simulink model "Simulate_FFNN"  (Simulink 10.2)
settings: Solver=ode45  StartTime=0.0  StopTime=10  RelTol=1e-3  EnableMultiTasking=on
libraries: slpidlib x22
settings Model: Creator=Administrator  LastModifiedBy=hunter
settings SolverCC: ZeroCrossControl=DisableAll
settings DataIOCC: LimitDataPoints=on
settings OptimizationCC: ExpressionDepthLimit=2147483647
settings DebuggingCC: SolverPrmCheckMsg=warning  StateNameClashWarn=warning

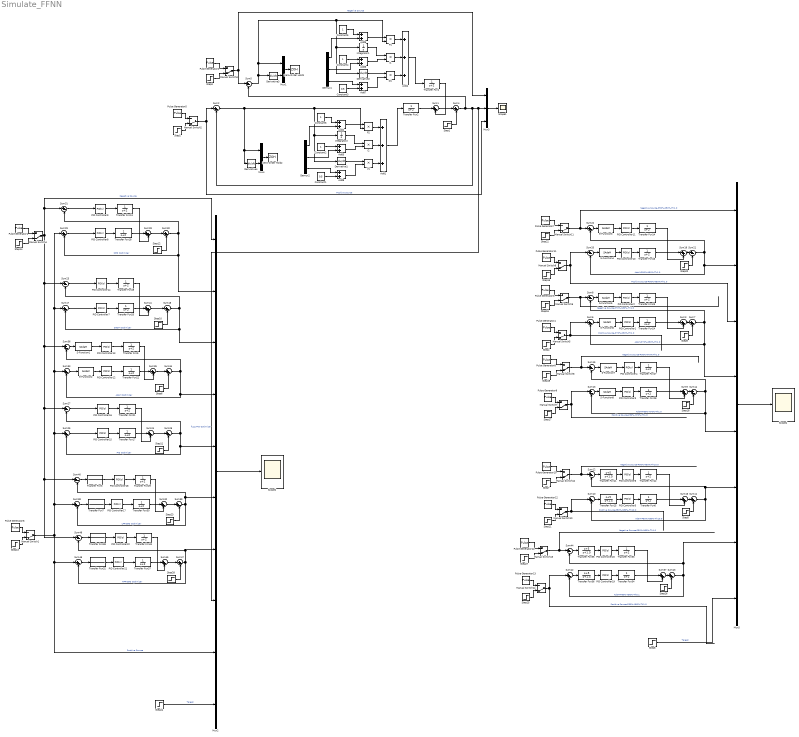
== system Simulate_FFNN ==
  Add1 : Sum  Inputs=+++
  Add{2..3,5..8} (6 alike) : Sum
  Add4 : Sum  Inputs=+++
  Constant1 : Constant  Value=0.5
  Constant{2,4..6} (4 alike) : Constant
  Constant3 : Constant  Value=0.5
  D1 : Product
  D2 : Product
  Demux1 : Demux  Outputs=3
  Demux2 : Demux  Outputs=3
  Derivative{1..4} (4 alike) : Derivative
  I1 : Product
  I2 : Product
  Integrator1 : Integrator
  Integrator2 : Integrator
  Manual Switch{1..14} (14 alike) : ManualSwitch  CurrentSetting=0
  Mux1 : Mux  Inputs=2
  Mux2 : Mux  Inputs=10
  Mux3 : Mux  Inputs=3
  Mux4 : Mux  Inputs=2
  Mux5 : Mux  Inputs=8
  P1 : Product
  P2 : Product
  PID Controller{1..4,8..13,17..18,21..22} (14 alike) : slpidlib/PID Controller  Controller=PID  Form=Parallel  TimeDomain=Continuous-time  UseExternalTs=off  SampleTime=-1  IntegratorMethod=Forward Euler  FilterMethod=Forward Euler  ControllerParametersSource=internal  P=1  I=0  D=0  UseFilter=on  N=100  TunerSelectOption=Transfer Function Based (PID Tuner App)  InitialConditionSource=internal  InitialConditionForIntegrator=0  InitialConditionForFilter=0  DifferentiatorICPrevScaledInput=0  ExternalReset=none  TrackingMode=off  Kt=1  LimitOutput=off  SatLimitsSource=internal  UpperSaturationLimit=inf  LowerSaturationLimit=-inf  LinearizeAsGain=on  AntiWindupMode=none  Kb=1  POutMin=[]  POutMax=[]  IOutMin=[]  IOutMax=[]  DOutMin=[]  DOutMax=[]  NOutMin=[]  NOutMax=[]  SumOutMin=[]  SumOutMax=[]  SaturationOutMin=[]  SaturationOutMax=[]  PParamMin=[]  PParamMax=[]  IParamMin=[]  IParamMax=[]  DParamMin=[]  DParamMax=[]  NParamMin=[]  NParamMax=[]  KbParamMin=[]  KbParamMax=[]  KtParamMin=[]  KtParamMax=[]  KbOutMin=[]  KbOutMax=[]  KtOutMin=[]  KtOutMax=[]  IntegratorOutMin=[]  IntegratorOutMax=[]  FilterOutMin=[]  FilterOutMax=[]  SumI1OutMin=[]  SumI1OutMax=[]  SumI2OutMin=[]  SumI2OutMax=[]  SumI3OutMin=[]  SumI3OutMax=[]  SumI4OutMin=[]  SumI4OutMax=[]  SumDOutMin=[]  SumDOutMax=[]  DifferentiatorOutMin=[]  DifferentiatorOutMax=[]  FilterDiffOutCoefMin=[]  FilterDiffOutCoefMax=[]  ReciprocalOutMin=[]  ReciprocalOutMax=[]  SumDenOutMin=[]  SumDenOutMax=[]  SumNumOutMin=[]  SumNumOutMax=[]  DivideOutMin=[]  DivideOutMax=[]  UdiffTsProdOutMin=[]  UdiffTsProdOutMax=[]  NTsProdOutMin=[]  NTsProdOutMax=[]  UintegralTsProdOutMin=[]  UintegralTsProdOutMax=[]  UngainTsProdOutMin=[]  UngainTsProdOutMax=[]  IntegratorContinuousStateAttributes=''  IntegratorStateMustResolveToSignalObject=off  IntegratorRTWStateStorageClass=Auto  FilterContinuousStateAttributes=''  FilterStateMustResolveToSignalObject=off  FilterRTWStateStorageClass=Auto  ParallelPVariant=InternalParameters  IdealPVariant=Disabled  IVariant=InternalParameters  DVariant=InternalParameters  IntegratorVariant=Continuous  SatVariant=Disabled  AWVariant=Passthrough  PCopyVariant=Disabled  TRVariant=Disabled  FdbkBlocksVariant=Forward  IdealPFdbkVariant=Disabled  SatFdbkVariant=Disabled  DerivativeFilterVariant=ContFilter  NVariant=InternalParameters  NCopyVariant=Disabled  FilterICVariant=InternalICsFilter  IntegratorICVariant=InternalICs  ExternalResetVariant=Disabled  TRSumVariant=Passthrough  SumFdbkVariant=Disabled  SumVariant=Sum_PID  TsampFilterVariant=InternalTs  TsampNgainVariant=Passthrough  TsampIntegralVariant=Passthrough  ExternalSaturationOutDataTypeStr=Inherit: Same as second input
  PID Controller{5..7,14,19..20} (6 alike) : slpidlib/PID Controller  Controller=PID  Form=Parallel  TimeDomain=Continuous-time  UseExternalTs=off  SampleTime=-1  IntegratorMethod=Forward Euler  FilterMethod=Forward Euler  ControllerParametersSource=internal  P=1  I=1  D=0  UseFilter=on  N=100  TunerSelectOption=Transfer Function Based (PID Tuner App)  InitialConditionSource=internal  InitialConditionForIntegrator=0  InitialConditionForFilter=0  DifferentiatorICPrevScaledInput=0  ExternalReset=none  TrackingMode=off  Kt=1  LimitOutput=off  SatLimitsSource=internal  UpperSaturationLimit=inf  LowerSaturationLimit=-inf  LinearizeAsGain=on  AntiWindupMode=none  Kb=1  POutMin=[]  POutMax=[]  IOutMin=[]  IOutMax=[]  DOutMin=[]  DOutMax=[]  NOutMin=[]  NOutMax=[]  SumOutMin=[]  SumOutMax=[]  SaturationOutMin=[]  SaturationOutMax=[]  PParamMin=[]  PParamMax=[]  IParamMin=[]  IParamMax=[]  DParamMin=[]  DParamMax=[]  NParamMin=[]  NParamMax=[]  KbParamMin=[]  KbParamMax=[]  KtParamMin=[]  KtParamMax=[]  KbOutMin=[]  KbOutMax=[]  KtOutMin=[]  KtOutMax=[]  IntegratorOutMin=[]  IntegratorOutMax=[]  FilterOutMin=[]  FilterOutMax=[]  SumI1OutMin=[]  SumI1OutMax=[]  SumI2OutMin=[]  SumI2OutMax=[]  SumI3OutMin=[]  SumI3OutMax=[]  SumI4OutMin=[]  SumI4OutMax=[]  SumDOutMin=[]  SumDOutMax=[]  DifferentiatorOutMin=[]  DifferentiatorOutMax=[]  FilterDiffOutCoefMin=[]  FilterDiffOutCoefMax=[]  ReciprocalOutMin=[]  ReciprocalOutMax=[]  SumDenOutMin=[]  SumDenOutMax=[]  SumNumOutMin=[]  SumNumOutMax=[]  DivideOutMin=[]  DivideOutMax=[]  UdiffTsProdOutMin=[]  UdiffTsProdOutMax=[]  NTsProdOutMin=[]  NTsProdOutMax=[]  UintegralTsProdOutMin=[]  UintegralTsProdOutMax=[]  UngainTsProdOutMin=[]  UngainTsProdOutMax=[]  IntegratorContinuousStateAttributes=''  IntegratorStateMustResolveToSignalObject=off  IntegratorRTWStateStorageClass=Auto  FilterContinuousStateAttributes=''  FilterStateMustResolveToSignalObject=off  FilterRTWStateStorageClass=Auto  ParallelPVariant=InternalParameters  IdealPVariant=Disabled  IVariant=InternalParameters  DVariant=InternalParameters  IntegratorVariant=Continuous  SatVariant=Disabled  AWVariant=Passthrough  PCopyVariant=Disabled  TRVariant=Disabled  FdbkBlocksVariant=Forward  IdealPFdbkVariant=Disabled  SatFdbkVariant=Disabled  DerivativeFilterVariant=ContFilter  NVariant=InternalParameters  NCopyVariant=Disabled  FilterICVariant=InternalICsFilter  IntegratorICVariant=InternalICs  ExternalResetVariant=Disabled  TRSumVariant=Passthrough  SumFdbkVariant=Disabled  SumVariant=Sum_PID  TsampFilterVariant=InternalTs  TsampNgainVariant=Passthrough  TsampIntegralVariant=Passthrough  ExternalSaturationOutDataTypeStr=Inherit: Same as second input
  PID Controller15 : slpidlib/PID Controller  Controller=PID  Form=Parallel  TimeDomain=Continuous-time  UseExternalTs=off  SampleTime=-1  IntegratorMethod=Forward Euler  FilterMethod=Forward Euler  ControllerParametersSource=internal  P=1  I=1.1  D=0.1  UseFilter=on  N=100  TunerSelectOption=Transfer Function Based (PID Tuner App)  InitialConditionSource=internal  InitialConditionForIntegrator=0  InitialConditionForFilter=0  DifferentiatorICPrevScaledInput=0  ExternalReset=none  TrackingMode=off  Kt=1  LimitOutput=off  SatLimitsSource=internal  UpperSaturationLimit=inf  LowerSaturationLimit=-inf  LinearizeAsGain=on  AntiWindupMode=none  Kb=1  POutMin=[]  POutMax=[]  IOutMin=[]  IOutMax=[]  DOutMin=[]  DOutMax=[]  NOutMin=[]  NOutMax=[]  SumOutMin=[]  SumOutMax=[]  SaturationOutMin=[]  SaturationOutMax=[]  PParamMin=[]  PParamMax=[]  IParamMin=[]  IParamMax=[]  DParamMin=[]  DParamMax=[]  NParamMin=[]  NParamMax=[]  KbParamMin=[]  KbParamMax=[]  KtParamMin=[]  KtParamMax=[]  KbOutMin=[]  KbOutMax=[]  KtOutMin=[]  KtOutMax=[]  IntegratorOutMin=[]  IntegratorOutMax=[]  FilterOutMin=[]  FilterOutMax=[]  SumI1OutMin=[]  SumI1OutMax=[]  SumI2OutMin=[]  SumI2OutMax=[]  SumI3OutMin=[]  SumI3OutMax=[]  SumI4OutMin=[]  SumI4OutMax=[]  SumDOutMin=[]  SumDOutMax=[]  DifferentiatorOutMin=[]  DifferentiatorOutMax=[]  FilterDiffOutCoefMin=[]  FilterDiffOutCoefMax=[]  ReciprocalOutMin=[]  ReciprocalOutMax=[]  SumDenOutMin=[]  SumDenOutMax=[]  SumNumOutMin=[]  SumNumOutMax=[]  DivideOutMin=[]  DivideOutMax=[]  UdiffTsProdOutMin=[]  UdiffTsProdOutMax=[]  NTsProdOutMin=[]  NTsProdOutMax=[]  UintegralTsProdOutMin=[]  UintegralTsProdOutMax=[]  UngainTsProdOutMin=[]  UngainTsProdOutMax=[]  IntegratorContinuousStateAttributes=''  IntegratorStateMustResolveToSignalObject=off  IntegratorRTWStateStorageClass=Auto  FilterContinuousStateAttributes=''  FilterStateMustResolveToSignalObject=off  FilterRTWStateStorageClass=Auto  ParallelPVariant=InternalParameters  IdealPVariant=Disabled  IVariant=InternalParameters  DVariant=InternalParameters  IntegratorVariant=Continuous  SatVariant=Disabled  AWVariant=Passthrough  PCopyVariant=Disabled  TRVariant=Disabled  FdbkBlocksVariant=Forward  IdealPFdbkVariant=Disabled  SatFdbkVariant=Disabled  DerivativeFilterVariant=ContFilter  NVariant=InternalParameters  NCopyVariant=Disabled  FilterICVariant=InternalICsFilter  IntegratorICVariant=InternalICs  ExternalResetVariant=Disabled  TRSumVariant=Passthrough  SumFdbkVariant=Disabled  SumVariant=Sum_PID  TsampFilterVariant=InternalTs  TsampNgainVariant=Passthrough  TsampIntegralVariant=Passthrough  ExternalSaturationOutDataTypeStr=Inherit: Same as second input
  PID Controller16 : slpidlib/PID Controller  Controller=PID  Form=Parallel  TimeDomain=Continuous-time  UseExternalTs=off  SampleTime=-1  IntegratorMethod=Forward Euler  FilterMethod=Forward Euler  ControllerParametersSource=internal  P=1  I=1.1  D=0.1  UseFilter=on  N=100  TunerSelectOption=Transfer Function Based (PID Tuner App)  InitialConditionSource=internal  InitialConditionForIntegrator=0  InitialConditionForFilter=0  DifferentiatorICPrevScaledInput=0  ExternalReset=none  TrackingMode=off  Kt=1  LimitOutput=off  SatLimitsSource=internal  UpperSaturationLimit=inf  LowerSaturationLimit=-inf  LinearizeAsGain=on  AntiWindupMode=none  Kb=1  POutMin=[]  POutMax=[]  IOutMin=[]  IOutMax=[]  DOutMin=[]  DOutMax=[]  NOutMin=[]  NOutMax=[]  SumOutMin=[]  SumOutMax=[]  SaturationOutMin=[]  SaturationOutMax=[]  PParamMin=[]  PParamMax=[]  IParamMin=[]  IParamMax=[]  DParamMin=[]  DParamMax=[]  NParamMin=[]  NParamMax=[]  KbParamMin=[]  KbParamMax=[]  KtParamMin=[]  KtParamMax=[]  KbOutMin=[]  KbOutMax=[]  KtOutMin=[]  KtOutMax=[]  IntegratorOutMin=[]  IntegratorOutMax=[]  FilterOutMin=[]  FilterOutMax=[]  SumI1OutMin=[]  SumI1OutMax=[]  SumI2OutMin=[]  SumI2OutMax=[]  SumI3OutMin=[]  SumI3OutMax=[]  SumI4OutMin=[]  SumI4OutMax=[]  SumDOutMin=[]  SumDOutMax=[]  DifferentiatorOutMin=[]  DifferentiatorOutMax=[]  FilterDiffOutCoefMin=[]  FilterDiffOutCoefMax=[]  ReciprocalOutMin=[]  ReciprocalOutMax=[]  SumDenOutMin=[]  SumDenOutMax=[]  SumNumOutMin=[]  SumNumOutMax=[]  DivideOutMin=[]  DivideOutMax=[]  UdiffTsProdOutMin=[]  UdiffTsProdOutMax=[]  NTsProdOutMin=[]  NTsProdOutMax=[]  UintegralTsProdOutMin=[]  UintegralTsProdOutMax=[]  UngainTsProdOutMin=[]  UngainTsProdOutMax=[]  IntegratorContinuousStateAttributes=''  IntegratorStateMustResolveToSignalObject=off  IntegratorRTWStateStorageClass=Auto  FilterContinuousStateAttributes=''  FilterStateMustResolveToSignalObject=off  FilterRTWStateStorageClass=Auto  ParallelPVariant=InternalParameters  IdealPVariant=Disabled  IVariant=InternalParameters  DVariant=InternalParameters  IntegratorVariant=Continuous  SatVariant=Disabled  AWVariant=Passthrough  PCopyVariant=Disabled  TRVariant=Disabled  FdbkBlocksVariant=Forward  IdealPFdbkVariant=Disabled  SatFdbkVariant=Disabled  DerivativeFilterVariant=ContFilter  NVariant=InternalParameters  NCopyVariant=Disabled  FilterICVariant=InternalICsFilter  IntegratorICVariant=InternalICs  ExternalResetVariant=Disabled  TRSumVariant=Passthrough  SumFdbkVariant=Disabled  SumVariant=Sum_PID  TsampFilterVariant=InternalTs  TsampNgainVariant=Passthrough  TsampIntegralVariant=Passthrough  ExternalSaturationOutDataTypeStr=Inherit: Same as second input
  Pulse Generator1 : DiscretePulseGenerator  PulseType=Time based  Period=40  PulseWidth=50  PhaseDelay=20
  Pulse Generator{3,7..8,10,14} (5 alike) : DiscretePulseGenerator  PulseType=Time based  Amplitude=-0.1  Period=20  PulseWidth=50
  Pulse Generator{4,9,11..13} (5 alike) : DiscretePulseGenerator  PulseType=Time based  Amplitude=0.1  Period=20  PulseWidth=50
  Pulse Generator2 : DiscretePulseGenerator  PulseType=Time based  Period=40  PulseWidth=50  PhaseDelay=20
  Pulse Generator5 : DiscretePulseGenerator  PulseType=Time based  Period=40  PulseWidth=50
  Pulse Generator6 : DiscretePulseGenerator  PulseType=Time based  Period=40  PulseWidth=50
  S-Function{1..8} (8 alike) : S-Function  FunctionName=SAdaM  SFunctionDeploymentMode=off  EnableBusSupport=off
  Scope1 : Scope
  Scope2 : Scope
  Scope4 : Scope
  Step{1,6,9..12,18,20,23,28} (10 alike) : Step  Time=0  SampleTime=0
  Step{2,13,15,21,25} (5 alike) : Step  Time=0  After=0.5  SampleTime=0
  Step{3,7,14,22,27} (5 alike) : Step  Time=0  After=-0.5  SampleTime=0
  Step16 : Step  Time=0  After=-0.3  SampleTime=0
  Step17 : Step  Time=0  After=0.3  SampleTime=0
  Step19 : Step  Time=0  After=-0.7  SampleTime=0
  Step24 : Step  Time=0  After=0  SampleTime=0
  Step26 : Step  Time=0  After=0.1  SampleTime=0
  Step4 : Step  Time=0  After=0.7  SampleTime=0
  Step5 : Step  Time=0  After=3  SampleTime=0
  Step8 : Step  Time=0  After=0  SampleTime=0
  Sum{1,3,9,16,19,24,28,32,35,37,41,45} (12 alike) : Sum  Inputs=|++
  Sum{2,4..8,10..15,17..18,20..23,25..27,29..31,33..34,36,38..40,42..44,46..48} (36 alike) : Sum  Inputs=|+-
  Transfer Fcn{1..2,5..6,12..14,16..24,27..31,33..34,37} (24 alike) : TransferFcn  Denominator=[1 2]
  Transfer Fcn{11,15,35..36} (4 alike) : TransferFcn  Numerator=[1 5]  Denominator=[1 1.5]
  Transfer Fcn3 : TransferFcn  Numerator=[0.01]  Denominator=[1 0.2 0.01]
  Transfer Fcn32 : TransferFcn  Numerator=[1 0.01]  Denominator=[1 0.2 0.01]
  Transfer Fcn38 : TransferFcn  Numerator=[1 0.01]  Denominator=[1 0.2 0.01]
  Transfer Fcn7 : TransferFcn  Numerator=[0.01]  Denominator=[1 0.2 0.01]
  Zero-Order Hold1 : ZeroOrderHold
  Zero-Order Hold2 : ZeroOrderHold
  wires:
  Step2/1 -> Manual Switch2/2
  Mux3/1 -> Scope1/1
  Step3/1 -> Manual Switch3/2
  Step1/1 -> Sum4/2
  Manual Switch2/1 -> Mux3/3, Sum2/1  "Positive Source"
  Pulse Generator5/1 -> Manual Switch2/1
  Manual Switch3/1 -> Sum5/1, Mux3/1  "Negative Source"
  Add1/1 -> Transfer Fcn2/1
  Transfer Fcn1/1 -> Sum1/2
  Pulse Generator2/1 -> Manual Switch3/1
  Add7/1 -> D1/2
  Sum5/1 -> Derivative3/1, Mux1/1, Derivative2/1, Integrator1/1, P1/2
  Derivative3/1 -> Mux1/2
  Integrator1/1 -> I1/1
  Mux1/1 -> Zero-Order Hold1/1
  D1/1 -> Add4/3
  P1/1 -> Add4/1
  Add4/1 -> Transfer Fcn1/1
  Demux1/2 -> Add6/2
  I1/1 -> Add4/2
  Constant5/1 -> Add5/1
  Constant4/1 -> Add6/1
  Constant3/1 -> Add7/2
  Demux1/3 -> Add7/1
  Derivative2/1 -> D1/1
  Demux1/1 -> Add5/2
  Add5/1 -> P1/1
  Add6/1 -> I1/2
  Add8/1 -> D2/2
  Sum2/1 -> Derivative1/1, Integrator2/1, P2/2, Derivative4/1, Mux4/1
  Derivative4/1 -> Mux4/2
  Integrator2/1 -> I2/1
  Mux4/1 -> Zero-Order Hold2/1
  D2/1 -> Add1/3
  P2/1 -> Add1/1
  Demux2/2 -> Add3/2
  I2/1 -> Add1/2
  Constant6/1 -> Add2/1
  Constant2/1 -> Add3/1
  Constant1/1 -> Add8/2
  Demux2/3 -> Add8/1
  Derivative1/1 -> D2/1
  Demux2/1 -> Add2/2
  Add2/1 -> P2/1
  Add3/1 -> I2/2
  PID Controller12/1 -> Transfer Fcn22/1
  Transfer Fcn5/1 -> Sum35/2
  Sum36/1 -> S-Function1/1
  Sum34/1 -> Sum33/2, Mux2/4, Sum36/2  "AdaM Optimizer"
  PID Controller13/1 -> Transfer Fcn5/1
  Step6/1 -> Sum34/2
  S-Function2/1 -> PID Controller12/1
  S-Function1/1 -> PID Controller13/1
  Sum18/1 -> Sum17/2, Mux2/3, Sum23/2  "SGDM Optimizer"
  Sum27/1 -> PID Controller16/1
  Sum23/1 -> PID Controller14/1
  Sum33/1 -> S-Function2/1
  Transfer Fcn21/1 -> Sum24/2
  PID Controller15/1 -> Transfer Fcn17/1
  PID Controller16/1 -> Transfer Fcn21/1
  Step10/1 -> Sum18/2
  Sum4/1 -> Sum2/2, Mux2/8, Mux3/2, Sum5/2  "fuzzyPID Optimizer"
  Sum17/1 -> PID Controller7/1
  Sum25/1 -> PID Controller15/1
  Transfer Fcn19/1 -> Sum41/2
  Step13/1 -> Manual Switch1/2
  Mux2/1 -> Scope2/1
  Step14/1 -> Manual Switch4/2
  Step12/1 -> Sum30/2
  Sum30/1 -> Sum29/2, Mux2/2, Sum31/2  "SGD Optimizer"
  Step11/1 -> Sum26/2
  PID Controller7/1 -> Transfer Fcn20/1
  Sum26/1 -> Sum25/2, Mux2/5, Sum27/2  "PID Optimizer"
  Pulse Generator6/1 -> Manual Switch1/1
  PID Controller9/1 -> Transfer Fcn13/1
  PID Controller8/1 -> Transfer Fcn18/1
  Transfer Fcn13/1 -> Sum28/2
  Sum31/1 -> PID Controller9/1
  Pulse Generator1/1 -> Manual Switch4/1
  Sum29/1 -> PID Controller8/1
  PID Controller14/1 -> Transfer Fcn19/1
  Pulse Generator9/1 -> Manual Switch7/1
  Sum9/1 -> Sum14/1
  Manual Switch7/1 -> Sum13/1  "Positive Source-P30%-N70%-Th1.0"
  Step18/1 -> Sum14/2
  Step19/1 -> Manual Switch8/2
  Manual Switch8/1 -> Sum15/1  "Negative Source-P30%-N70%-Th1.0"
  Sum14/1 -> Mux5/5, Sum13/2, Sum15/2  "AdaM-P30%-N70%-Th1.0"
  Transfer Fcn27/1 -> Sum9/2
  PID Controller4/1 -> Transfer Fcn27/1
  Pulse Generator8/1 -> Manual Switch8/1
  Transfer Fcn28/1 -> Sum9/1
  Pulse Generator4/1 -> Manual Switch5/1
  Step9/1 -> Sum7/2
  Manual Switch5/1 -> Sum6/1  "Positive Source-P70%-N30%-Th1.0"
  Sum3/1 -> Sum7/1
  Step4/1 -> Manual Switch5/2
  Step16/1 -> Manual Switch6/2
  Sum7/1 -> Sum6/2, Mux5/4, Sum8/2  "AdaM-P70%-N30%-Th1.0"
  Pulse Generator3/1 -> Manual Switch6/1
  Transfer Fcn14/1 -> Sum19/2
  Sum21/1 -> Mux5/2, Sum20/2, Sum22/2  "AdaM-P50%-N50%-Th1.0"
  Step22/1 -> Manual Switch11/2
  Manual Switch9/1 -> Mux5/3, Sum20/1  "Positive Source-P50%-N50%-Th1.0"
  Step15/1 -> Manual Switch9/2
  S-Function3/1 -> PID Controller11/1
  S-Function4/1 -> PID Controller10/1
  Sum12/1 -> Transfer Fcn11/1
  Sum10/1 -> Transfer Fcn15/1
  PID Controller5/1 -> Transfer Fcn6/1
  Pulse Generator12/1 -> Manual Switch10/1
  Step5/1 -> Sum11/2
  Sum16/1 -> Sum11/1
  Sum20/1 -> S-Function4/1
  Step7/1 -> Manual Switch12/2
  Manual Switch10/1 -> Sum10/1  "Positive Source-P50%-N50%-Th10.0"
  Pulse Generator7/1 -> Manual Switch11/1
  Transfer Fcn15/1 -> PID Controller5/1
  Sum11/1 -> Mux5/6, Sum12/2, Sum10/2  "AdaM-P50%-N50%-Th10.0"
  Transfer Fcn23/1 -> Sum3/2
  Step21/1 -> Manual Switch10/2
  Manual Switch12/1 -> Sum12/1  "Negative Source-P50%-N50%-Th10.0"
  PID Controller6/1 -> Transfer Fcn12/1
  Transfer Fcn12/1 -> Sum16/2
  Transfer Fcn6/1 -> Sum16/1
  Transfer Fcn16/1 -> Sum19/1
  Transfer Fcn11/1 -> PID Controller6/1
  Mux5/1 -> Scope4/1
  Sum19/1 -> Sum21/1
  Step20/1 -> Sum21/2
  PID Controller10/1 -> Transfer Fcn16/1
  Manual Switch6/1 -> Sum8/1  "Negative Source-P70%-N30%-Th1.0"
  Sum22/1 -> S-Function3/1
  Transfer Fcn24/1 -> Sum3/1
  Step8/1 -> Mux5/8  "Target"
  PID Controller11/1 -> Transfer Fcn14/1
  Pulse Generator10/1 -> Manual Switch12/1
  Step17/1 -> Manual Switch7/2
  Manual Switch11/1 -> Mux5/1, Sum22/1  "Negative Source-P50%-N50%-Th1.0"
  Pulse Generator11/1 -> Manual Switch9/1
  Transfer Fcn18/1 -> Sum28/1
  Sum28/1 -> Sum30/1
  Transfer Fcn20/1 -> Sum41/1
  Sum41/1 -> Sum18/1
  Transfer Fcn22/1 -> Sum35/1
  Sum35/1 -> Sum34/1
  Transfer Fcn17/1 -> Sum24/1
  Sum24/1 -> Sum26/1
  Transfer Fcn2/1 -> Sum1/1
  Sum1/1 -> Sum4/1
  Step24/1 -> Mux2/10  "Target"
  Sum37/1 -> Sum43/1
  Pulse Generator13/1 -> Manual Switch14/1
  Transfer Fcn33/1 -> Sum37/2
  Pulse Generator14/1 -> Manual Switch13/1
  PID Controller20/1 -> Transfer Fcn33/1
  Sum44/1 -> Transfer Fcn35/1
  Step25/1 -> Manual Switch14/2
  Transfer Fcn35/1 -> PID Controller20/1
  Transfer Fcn36/1 -> PID Controller19/1
  Sum42/1 -> Transfer Fcn36/1
  Manual Switch14/1 -> Sum42/1  "Positive Source-P50%-N50%-Th1.0"
  Step27/1 -> Manual Switch13/2
  Sum43/1 -> Mux5/7, Sum44/2, Sum42/2  "AdaM-P50%-N50%-Th0.1"
  Step26/1 -> Sum43/2
  Transfer Fcn34/1 -> Sum37/1
  Manual Switch13/1 -> Sum44/1  "Negative Source-P50%-N50%-Th1.0"
  PID Controller19/1 -> Transfer Fcn34/1
  Transfer Fcn30/1 -> Sum32/1
  PID Controller18/1 -> Transfer Fcn29/1
  Sum40/1 -> Transfer Fcn3/1
  Sum39/1 -> Mux2/6, Sum40/2, Sum38/2  "LPF-SGD Optimizer"
  Step23/1 -> Sum39/2
  Transfer Fcn7/1 -> PID Controller17/1
  Transfer Fcn3/1 -> PID Controller18/1
  Transfer Fcn29/1 -> Sum32/2
  Sum38/1 -> Transfer Fcn7/1
  PID Controller17/1 -> Transfer Fcn30/1
  Sum32/1 -> Sum39/1
  Transfer Fcn38/1 -> PID Controller22/1
  Sum45/1 -> Sum47/1
  PID Controller21/1 -> Transfer Fcn37/1
  Transfer Fcn32/1 -> PID Controller21/1
  Transfer Fcn31/1 -> Sum45/2
  Step28/1 -> Sum47/2
  Manual Switch4/1 -> Mux2/1, Sum31/1, Sum23/1, Sum36/1, Sum27/1, Sum48/1, Sum40/1  "Negative Source"
  Transfer Fcn37/1 -> Sum45/1
  Sum48/1 -> Transfer Fcn38/1
  Sum47/1 -> Mux2/7, Sum48/2, Sum46/2  "HPF-SGD Optimizer"
  Sum46/1 -> Transfer Fcn32/1
  Manual Switch1/1 -> Mux2/9, Sum46/1, Sum38/1, Sum29/1, Sum17/1, Sum33/1, Sum25/1  "Positive Source"
  PID Controller22/1 -> Transfer Fcn31/1
  PID Controller2/1 -> Transfer Fcn23/1
  S-Function5/1 -> PID Controller2/1
  Sum8/1 -> S-Function5/1
  PID Controller1/1 -> Transfer Fcn24/1
  S-Function6/1 -> PID Controller1/1
  Sum6/1 -> S-Function6/1
  S-Function7/1 -> PID Controller4/1
  Sum15/1 -> S-Function7/1
  PID Controller3/1 -> Transfer Fcn28/1
  S-Function8/1 -> PID Controller3/1
  Sum13/1 -> S-Function8/1
